simulink model "simulasi_dual-axis tracker"  (R2022b)
settings: Solver=VariableStepAuto  StartTime=0.0  StopTime=20  RelTol=1e-3
values from neighbouring files (symbols this model uses):
  a = Cx/Ap    (= 93255.7445539)    [parameter.m]
  b = 1/(W)^2    (= 0.000296140802632)    [parameter.m]
  c = 2*z/W    (= 0.057133023576)    [parameter.m]
  d = 1    [parameter.m]    (also in sun_calculation.m = datetime('now','TimeZone','UTC+7','Format','dd/MM/yyyy HH:mm)
  k = 150    [parameter.m]
  Kc = 1.3    [parameter.m]
  L = 0.98    [parameter.m]
  m = 0.01    [parameter.m]
  R = 230.77    [parameter.m]
libraries: fuzblock x16
settings Model: Creator=HP  LastModifiedBy=HP

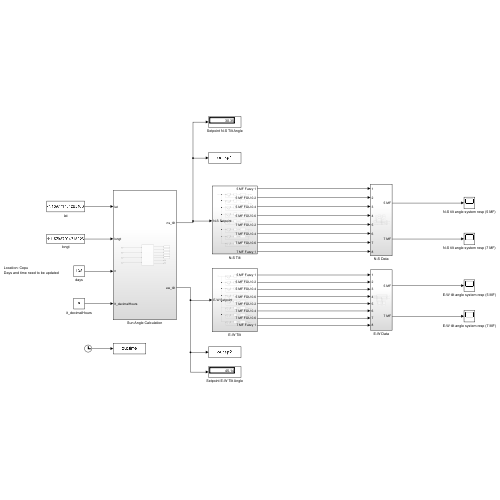
[thumbnail: Simulink's stored preview of the top-level diagram]
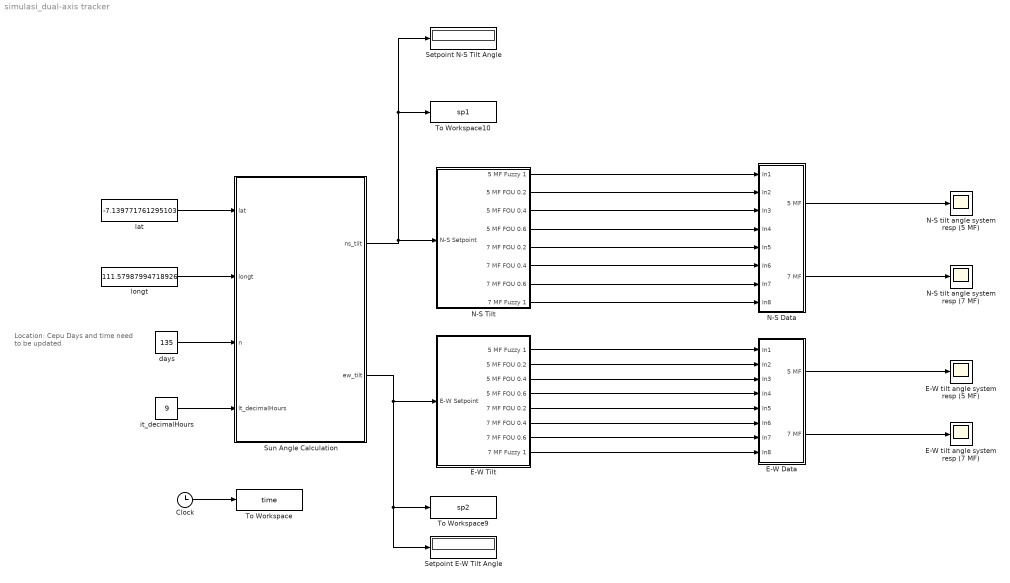
== system simulasi_dual-axis tracker ==
  note: Location: Cepu
      | Days and time need to be updated
  Clock : Clock
  E-W Data : Subsystem
  E-W Tilt : Subsystem
  E-W tilt angle system resp (5 MF) : Scope
  E-W tilt angle system resp (7 MF) : Scope
  N-S Data : Subsystem
  N-S Tilt : Subsystem
  N-S tilt angle system resp (5 MF) : Scope
  N-S tilt angle system resp (7 MF) : Scope
  Setpoint E-W Tilt Angle : Display
  Setpoint N-S Tilt Angle : Display
  Sun Angle Calculation : Subsystem
  To Workspace : ToWorkspace  VariableName=time  SampleTime=-1
  To Workspace10 : ToWorkspace  VariableName=sp1  SampleTime=-1
  To Workspace9 : ToWorkspace  VariableName=sp2  SampleTime=-1
  days : Constant  Value=135
  it_decimalHours : Constant  Value=9
  lat : Constant  Value=-7.139771761295103
  longt : Constant  Value=111.57987994718926
  wires:
  days/1 -> Sun Angle Calculation/3(n)
  longt/1 -> Sun Angle Calculation/2(longt)
  lat/1 -> Sun Angle Calculation/1(lat)
  it_decimalHours/1 -> Sun Angle Calculation/4(lt_decimalHours)
  Clock/1 -> To Workspace/1
  Sun Angle Calculation/1(ns_tilt) -> To Workspace10/1, Setpoint N-S Tilt Angle/1, N-S Tilt/1(N-S Setpoint)
  Sun Angle Calculation/2(ew_tilt) -> E-W Tilt/1(E-W Setpoint), Setpoint E-W Tilt Angle/1, To Workspace9/1
  E-W Tilt/1(5 MF Fuzzy 1) -> E-W Data/1(In1)
  E-W Tilt/2(5 MF FOU 0.2) -> E-W Data/2(In2)
  E-W Tilt/3(5 MF FOU 0.4) -> E-W Data/3(In3)
  E-W Tilt/4(5 MF FOU 0.6) -> E-W Data/4(In4)
  E-W Tilt/5(7 MF FOU 0.2) -> E-W Data/5(In5)
  E-W Tilt/6(7 MF FOU 0.4) -> E-W Data/6(In6)
  E-W Tilt/7(7 MF FOU 0.6) -> E-W Data/7(In7)
  E-W Tilt/8(7 MF Fuzzy 1) -> E-W Data/8(In8)
  E-W Data/1(5 MF) -> E-W tilt angle system resp (5 MF)/1
  E-W Data/2(7 MF) -> E-W tilt angle system resp (7 MF)/1
  N-S Tilt/1(5 MF Fuzzy 1) -> N-S Data/1(In1)
  N-S Tilt/2(5 MF FOU 0.2) -> N-S Data/2(In2)
  N-S Tilt/3(5 MF FOU 0.4) -> N-S Data/3(In3)
  N-S Tilt/4(5 MF FOU 0.6) -> N-S Data/4(In4)
  N-S Tilt/5(7 MF FOU 0.2) -> N-S Data/5(In5)
  N-S Tilt/6(7 MF FOU 0.4) -> N-S Data/6(In6)
  N-S Tilt/7(7 MF FOU 0.6) -> N-S Data/7(In7)
  N-S Tilt/8(7 MF Fuzzy 1) -> N-S Data/8(In8)
  N-S Data/1(5 MF) -> N-S tilt angle system resp (5 MF)/1
  N-S Data/2(7 MF) -> N-S tilt angle system resp (7 MF)/1

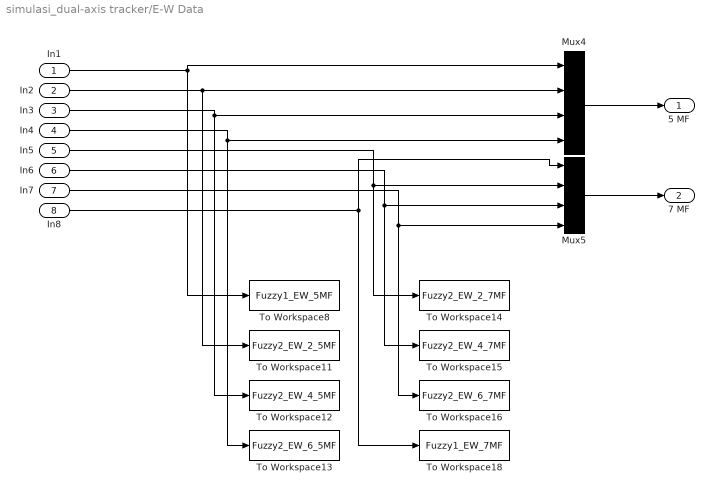
== system simulasi_dual-axis tracker/E-W Data ==
  In1 : Inport
  In2 : Inport  Port=2
  In3 : Inport  Port=3
  In4 : Inport  Port=4
  In5 : Inport  Port=5
  In6 : Inport  Port=6
  In7 : Inport  Port=7
  In8 : Inport  Port=8
  Mux4 : Mux
  Mux5 : Mux
  To Workspace11 : ToWorkspace  VariableName=Fuzzy2_EW_2_5MF  SampleTime=-1
  To Workspace12 : ToWorkspace  VariableName=Fuzzy2_EW_4_5MF  SampleTime=-1
  To Workspace13 : ToWorkspace  VariableName=Fuzzy2_EW_6_5MF  SampleTime=-1
  To Workspace14 : ToWorkspace  VariableName=Fuzzy2_EW_2_7MF  SampleTime=-1
  To Workspace15 : ToWorkspace  VariableName=Fuzzy2_EW_4_7MF  SampleTime=-1
  To Workspace16 : ToWorkspace  VariableName=Fuzzy2_EW_6_7MF  SampleTime=-1
  To Workspace18 : ToWorkspace  VariableName=Fuzzy1_EW_7MF  SampleTime=-1
  To Workspace8 : ToWorkspace  VariableName=Fuzzy1_EW_5MF  SampleTime=-1
  5 MF : Outport
  7 MF : Outport  Port=2
  wires:
  In7/1 -> To Workspace16/1, Mux5/4
  In4/1 -> To Workspace13/1, Mux4/4
  In6/1 -> To Workspace15/1, Mux5/3
  In1/1 -> Mux4/1, To Workspace8/1
  In8/1 -> Mux5/1, To Workspace18/1
  In2/1 -> To Workspace11/1, Mux4/2
  In5/1 -> To Workspace14/1, Mux5/2
  In3/1 -> To Workspace12/1, Mux4/3
  Mux4/1 -> 5 MF/1
  Mux5/1 -> 7 MF/1

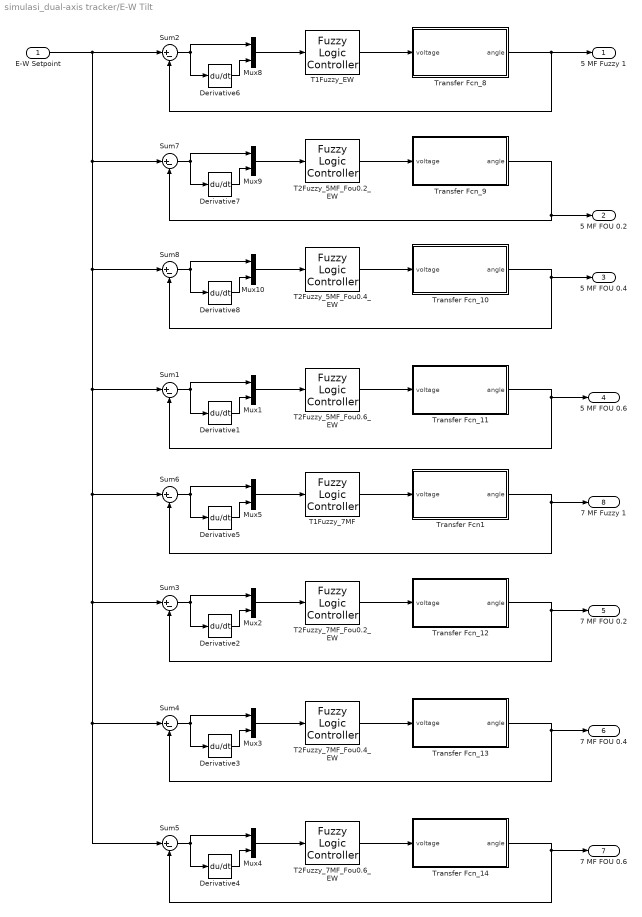
== system simulasi_dual-axis tracker/E-W Tilt ==
  E-W Setpoint : Inport
  Derivative{1..8} (8 alike) : Derivative
  Mux{1..5,8..10} (8 alike) : Mux  Inputs=2
  Sum{1..8} (8 alike) : Sum  Inputs=|+-
  T1Fuzzy_7MF : fuzblock/Fuzzy Logic  Controller  FIS='7mf_type1.fis'  OutputSampleNumber=101  DataType=double  FuzzifiedInputs=off  RuleFiringStrengths=off  RuleOutputs=off  AggregatedOutputs=off  SimulateUsing=Interpreted execution  OutOfRangeInputValueMessage=warning  NoRuleFiredMessage=warning  EmptyOutputFuzzySetMessage=warning
  T1Fuzzy_EW : fuzblock/Fuzzy Logic  Controller  FIS='5mf_type1.fis'  OutputSampleNumber=101  DataType=double  FuzzifiedInputs=off  RuleFiringStrengths=off  RuleOutputs=off  AggregatedOutputs=off  SimulateUsing=Interpreted execution  OutOfRangeInputValueMessage=warning  NoRuleFiredMessage=warning  EmptyOutputFuzzySetMessage=warning
  T2Fuzzy_5MF_Fou0.2_EW : fuzblock/Fuzzy Logic  Controller  FIS='5mf_type2_fou0.2.fis'  OutputSampleNumber=101  DataType=double  FuzzifiedInputs=off  RuleFiringStrengths=off  RuleOutputs=off  AggregatedOutputs=off  SimulateUsing=Interpreted execution  OutOfRangeInputValueMessage=warning  NoRuleFiredMessage=warning  EmptyOutputFuzzySetMessage=warning
  T2Fuzzy_5MF_Fou0.4_EW : fuzblock/Fuzzy Logic  Controller  FIS='5mf_type2_fou0.4.fis'  OutputSampleNumber=101  DataType=double  FuzzifiedInputs=off  RuleFiringStrengths=off  RuleOutputs=off  AggregatedOutputs=off  SimulateUsing=Interpreted execution  OutOfRangeInputValueMessage=warning  NoRuleFiredMessage=warning  EmptyOutputFuzzySetMessage=warning
  T2Fuzzy_5MF_Fou0.6_EW : fuzblock/Fuzzy Logic  Controller  FIS='5mf_type2_fou0.6.fis'  OutputSampleNumber=101  DataType=double  FuzzifiedInputs=off  RuleFiringStrengths=off  RuleOutputs=off  AggregatedOutputs=off  SimulateUsing=Interpreted execution  OutOfRangeInputValueMessage=warning  NoRuleFiredMessage=warning  EmptyOutputFuzzySetMessage=warning
  T2Fuzzy_7MF_Fou0.2_EW : fuzblock/Fuzzy Logic  Controller  FIS='7mf_type2_fou0.2.fis'  OutputSampleNumber=101  DataType=double  FuzzifiedInputs=off  RuleFiringStrengths=off  RuleOutputs=off  AggregatedOutputs=off  SimulateUsing=Interpreted execution  OutOfRangeInputValueMessage=warning  NoRuleFiredMessage=warning  EmptyOutputFuzzySetMessage=warning
  T2Fuzzy_7MF_Fou0.4_EW : fuzblock/Fuzzy Logic  Controller  FIS='7mf_type2_fou0.4.fis'  OutputSampleNumber=101  DataType=double  FuzzifiedInputs=off  RuleFiringStrengths=off  RuleOutputs=off  AggregatedOutputs=off  SimulateUsing=Interpreted execution  OutOfRangeInputValueMessage=warning  NoRuleFiredMessage=warning  EmptyOutputFuzzySetMessage=warning
  T2Fuzzy_7MF_Fou0.6_EW : fuzblock/Fuzzy Logic  Controller  FIS='7mf_type2_fou0.6.fis'  OutputSampleNumber=101  DataType=double  FuzzifiedInputs=off  RuleFiringStrengths=off  RuleOutputs=off  AggregatedOutputs=off  SimulateUsing=Interpreted execution  OutOfRangeInputValueMessage=warning  NoRuleFiredMessage=warning  EmptyOutputFuzzySetMessage=warning
  Transfer Fcn1 : Subsystem
  Transfer Fcn_10 : Subsystem
  Transfer Fcn_11 : Subsystem
  Transfer Fcn_12 : Subsystem
  Transfer Fcn_13 : Subsystem
  Transfer Fcn_14 : Subsystem
  Transfer Fcn_8 : Subsystem
  Transfer Fcn_9 : Subsystem
  5 MF Fuzzy 1 : Outport
  5 MF FOU 0.2 : Outport  Port=2
  5 MF FOU 0.4 : Outport  Port=3
  5 MF FOU 0.6 : Outport  Port=4
  7 MF FOU 0.2 : Outport  Port=5
  7 MF FOU 0.4 : Outport  Port=6
  7 MF FOU 0.6 : Outport  Port=7
  7 MF Fuzzy 1 : Outport  Port=8
  wires:
  Sum7/1 -> Derivative7/1, Mux9/1
  Transfer Fcn_9/1(angle) -> 5 MF FOU 0.2/1, Sum7/2
  T2Fuzzy_5MF_Fou0.4_EW/1 -> Transfer Fcn_10/1(voltage)
  Transfer Fcn_10/1(angle) -> 5 MF FOU 0.4/1, Sum8/2
  Derivative7/1 -> Mux9/2
  Mux9/1 -> T2Fuzzy_5MF_Fou0.2_EW/1
  Mux10/1 -> T2Fuzzy_5MF_Fou0.4_EW/1
  Derivative6/1 -> Mux8/2
  Mux8/1 -> T1Fuzzy_EW/1
  Sum2/1 -> Derivative6/1, Mux8/1
  Sum8/1 -> Derivative8/1, Mux10/1
  Derivative8/1 -> Mux10/2
  T1Fuzzy_EW/1 -> Transfer Fcn_8/1(voltage)
  Transfer Fcn_8/1(angle) -> 5 MF Fuzzy 1/1, Sum2/2
  T2Fuzzy_5MF_Fou0.2_EW/1 -> Transfer Fcn_9/1(voltage)
  Derivative1/1 -> Mux1/2
  Sum1/1 -> Derivative1/1, Mux1/1
  Mux1/1 -> T2Fuzzy_5MF_Fou0.6_EW/1
  Transfer Fcn_11/1(angle) -> 5 MF FOU 0.6/1, Sum1/2
  T2Fuzzy_5MF_Fou0.6_EW/1 -> Transfer Fcn_11/1(voltage)
  Sum3/1 -> Derivative2/1, Mux2/1
  Mux2/1 -> T2Fuzzy_7MF_Fou0.2_EW/1
  Derivative2/1 -> Mux2/2
  T2Fuzzy_7MF_Fou0.2_EW/1 -> Transfer Fcn_12/1(voltage)
  Transfer Fcn_12/1(angle) -> 7 MF FOU 0.2/1, Sum3/2
  Mux3/1 -> T2Fuzzy_7MF_Fou0.4_EW/1
  Sum4/1 -> Derivative3/1, Mux3/1
  Transfer Fcn_13/1(angle) -> 7 MF FOU 0.4/1, Sum4/2
  Derivative3/1 -> Mux3/2
  T2Fuzzy_7MF_Fou0.4_EW/1 -> Transfer Fcn_13/1(voltage)
  T2Fuzzy_7MF_Fou0.6_EW/1 -> Transfer Fcn_14/1(voltage)
  Derivative4/1 -> Mux4/2
  Sum5/1 -> Derivative4/1, Mux4/1
  Transfer Fcn_14/1(angle) -> 7 MF FOU 0.6/1, Sum5/2
  Mux4/1 -> T2Fuzzy_7MF_Fou0.6_EW/1
  Transfer Fcn1/1(angle) -> 7 MF Fuzzy 1/1, Sum6/2
  E-W Setpoint/1 -> Sum6/1, Sum5/1, Sum4/1, Sum3/1, Sum1/1, Sum8/1, Sum7/1, Sum2/1
  Derivative5/1 -> Mux5/2
  Mux5/1 -> T1Fuzzy_7MF/1
  Sum6/1 -> Derivative5/1, Mux5/1
  T1Fuzzy_7MF/1 -> Transfer Fcn1/1(voltage)

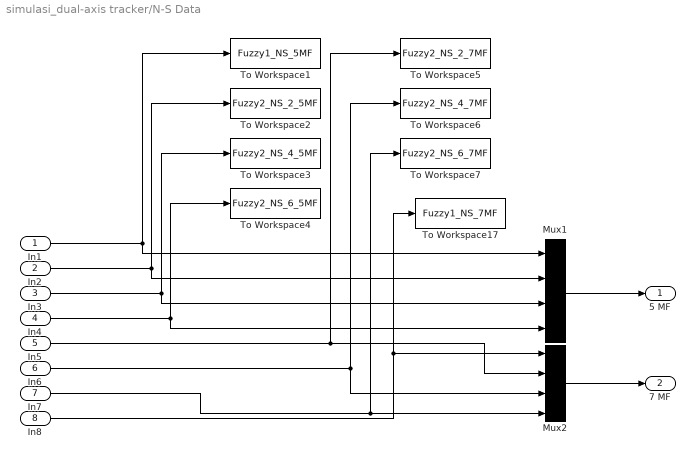
== system simulasi_dual-axis tracker/N-S Data ==
  In1 : Inport
  In2 : Inport  Port=2
  In3 : Inport  Port=3
  In4 : Inport  Port=4
  In5 : Inport  Port=5
  In6 : Inport  Port=6
  In7 : Inport  Port=7
  In8 : Inport  Port=8
  Mux1 : Mux
  Mux2 : Mux
  To Workspace1 : ToWorkspace  VariableName=Fuzzy1_NS_5MF  SampleTime=-1
  To Workspace17 : ToWorkspace  VariableName=Fuzzy1_NS_7MF  SampleTime=-1
  To Workspace2 : ToWorkspace  VariableName=Fuzzy2_NS_2_5MF  SampleTime=-1
  To Workspace3 : ToWorkspace  VariableName=Fuzzy2_NS_4_5MF  SampleTime=-1
  To Workspace4 : ToWorkspace  VariableName=Fuzzy2_NS_6_5MF  SampleTime=-1
  To Workspace5 : ToWorkspace  VariableName=Fuzzy2_NS_2_7MF  SampleTime=-1
  To Workspace6 : ToWorkspace  VariableName=Fuzzy2_NS_4_7MF  SampleTime=-1
  To Workspace7 : ToWorkspace  VariableName=Fuzzy2_NS_6_7MF  SampleTime=-1
  5 MF : Outport
  7 MF : Outport  Port=2
  wires:
  In8/1 -> To Workspace17/1, Mux2/1
  In2/1 -> Mux1/2, To Workspace2/1
  In5/1 -> Mux2/2, To Workspace5/1
  In6/1 -> Mux2/3, To Workspace6/1
  In3/1 -> Mux1/3, To Workspace3/1
  In4/1 -> Mux1/4, To Workspace4/1
  In7/1 -> To Workspace7/1, Mux2/4
  In1/1 -> Mux1/1, To Workspace1/1
  Mux1/1 -> 5 MF/1
  Mux2/1 -> 7 MF/1

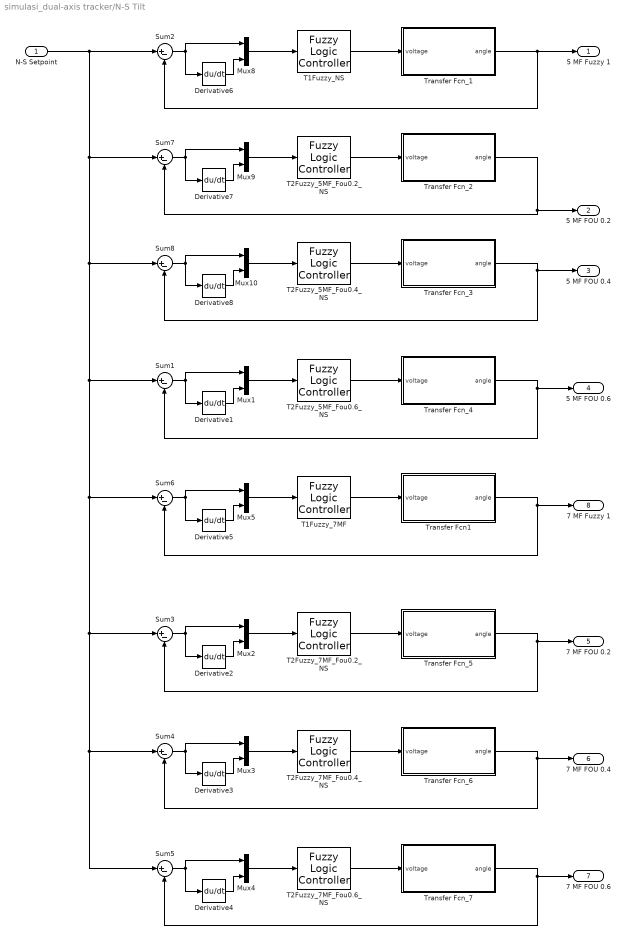
== system simulasi_dual-axis tracker/N-S Tilt ==
  N-S Setpoint : Inport
  Derivative{1..8} (8 alike) : Derivative
  Mux{1..5,8..10} (8 alike) : Mux  Inputs=2
  Sum{1..8} (8 alike) : Sum  Inputs=|+-
  T1Fuzzy_7MF : fuzblock/Fuzzy Logic  Controller  FIS='7mf_type1.fis'  OutputSampleNumber=101  DataType=double  FuzzifiedInputs=off  RuleFiringStrengths=off  RuleOutputs=off  AggregatedOutputs=off  SimulateUsing=Interpreted execution  OutOfRangeInputValueMessage=warning  NoRuleFiredMessage=warning  EmptyOutputFuzzySetMessage=warning
  T1Fuzzy_NS : fuzblock/Fuzzy Logic  Controller  FIS='5mf_type1.fis'  OutputSampleNumber=101  DataType=double  FuzzifiedInputs=off  RuleFiringStrengths=off  RuleOutputs=off  AggregatedOutputs=off  SimulateUsing=Interpreted execution  OutOfRangeInputValueMessage=warning  NoRuleFiredMessage=warning  EmptyOutputFuzzySetMessage=warning
  T2Fuzzy_5MF_Fou0.2_NS : fuzblock/Fuzzy Logic  Controller  FIS='5mf_type2_fou0.2.fis'  OutputSampleNumber=101  DataType=double  FuzzifiedInputs=off  RuleFiringStrengths=off  RuleOutputs=off  AggregatedOutputs=off  SimulateUsing=Interpreted execution  OutOfRangeInputValueMessage=warning  NoRuleFiredMessage=warning  EmptyOutputFuzzySetMessage=warning
  T2Fuzzy_5MF_Fou0.4_NS : fuzblock/Fuzzy Logic  Controller  FIS='5mf_type2_fou0.4.fis'  OutputSampleNumber=101  DataType=double  FuzzifiedInputs=off  RuleFiringStrengths=off  RuleOutputs=off  AggregatedOutputs=off  SimulateUsing=Interpreted execution  OutOfRangeInputValueMessage=warning  NoRuleFiredMessage=warning  EmptyOutputFuzzySetMessage=warning
  T2Fuzzy_5MF_Fou0.6_NS : fuzblock/Fuzzy Logic  Controller  FIS='5mf_type2_fou0.6.fis'  OutputSampleNumber=101  DataType=double  FuzzifiedInputs=off  RuleFiringStrengths=off  RuleOutputs=off  AggregatedOutputs=off  SimulateUsing=Interpreted execution  OutOfRangeInputValueMessage=warning  NoRuleFiredMessage=warning  EmptyOutputFuzzySetMessage=warning
  T2Fuzzy_7MF_Fou0.2_NS : fuzblock/Fuzzy Logic  Controller  FIS='7mf_type2_fou0.2.fis'  OutputSampleNumber=101  DataType=double  FuzzifiedInputs=off  RuleFiringStrengths=off  RuleOutputs=off  AggregatedOutputs=off  SimulateUsing=Interpreted execution  OutOfRangeInputValueMessage=warning  NoRuleFiredMessage=warning  EmptyOutputFuzzySetMessage=warning
  T2Fuzzy_7MF_Fou0.4_NS : fuzblock/Fuzzy Logic  Controller  FIS='7mf_type2_fou0.4.fis'  OutputSampleNumber=101  DataType=double  FuzzifiedInputs=off  RuleFiringStrengths=off  RuleOutputs=off  AggregatedOutputs=off  SimulateUsing=Interpreted execution  OutOfRangeInputValueMessage=warning  NoRuleFiredMessage=warning  EmptyOutputFuzzySetMessage=warning
  T2Fuzzy_7MF_Fou0.6_NS : fuzblock/Fuzzy Logic  Controller  FIS='7mf_type2_fou0.6.fis'  OutputSampleNumber=101  DataType=double  FuzzifiedInputs=off  RuleFiringStrengths=off  RuleOutputs=off  AggregatedOutputs=off  SimulateUsing=Interpreted execution  OutOfRangeInputValueMessage=warning  NoRuleFiredMessage=warning  EmptyOutputFuzzySetMessage=warning
  Transfer Fcn1 : Subsystem
  Transfer Fcn_1 : Subsystem
  Transfer Fcn_2 : Subsystem
  Transfer Fcn_3 : Subsystem
  Transfer Fcn_4 : Subsystem
  Transfer Fcn_5 : Subsystem
  Transfer Fcn_6 : Subsystem
  Transfer Fcn_7 : Subsystem
  5 MF Fuzzy 1 : Outport
  5 MF FOU 0.2 : Outport  Port=2
  5 MF FOU 0.4 : Outport  Port=3
  5 MF FOU 0.6 : Outport  Port=4
  7 MF FOU 0.2 : Outport  Port=5
  7 MF FOU 0.4 : Outport  Port=6
  7 MF FOU 0.6 : Outport  Port=7
  7 MF Fuzzy 1 : Outport  Port=8
  wires:
  Derivative3/1 -> Mux3/2
  Transfer Fcn_4/1(angle) -> 5 MF FOU 0.6/1, Sum1/2
  Transfer Fcn_7/1(angle) -> 7 MF FOU 0.6/1, Sum5/2
  T2Fuzzy_7MF_Fou0.6_NS/1 -> Transfer Fcn_7/1(voltage)
  Mux4/1 -> T2Fuzzy_7MF_Fou0.6_NS/1
  Derivative8/1 -> Mux10/2
  Transfer Fcn_3/1(angle) -> 5 MF FOU 0.4/1, Sum8/2
  Derivative2/1 -> Mux2/2
  Sum7/1 -> Derivative7/1, Mux9/1
  Sum3/1 -> Derivative2/1, Mux2/1
  Transfer Fcn_1/1(angle) -> 5 MF Fuzzy 1/1, Sum2/2
  Mux9/1 -> T2Fuzzy_5MF_Fou0.2_NS/1
  Mux2/1 -> T2Fuzzy_7MF_Fou0.2_NS/1
  Sum5/1 -> Derivative4/1, Mux4/1
  T2Fuzzy_5MF_Fou0.6_NS/1 -> Transfer Fcn_4/1(voltage)
  Derivative6/1 -> Mux8/2
  Sum2/1 -> Derivative6/1, Mux8/1
  Sum8/1 -> Derivative8/1, Mux10/1
  T2Fuzzy_5MF_Fou0.2_NS/1 -> Transfer Fcn_2/1(voltage)
  Transfer Fcn_5/1(angle) -> 7 MF FOU 0.2/1, Sum3/2
  Sum1/1 -> Derivative1/1, Mux1/1
  Mux3/1 -> T2Fuzzy_7MF_Fou0.4_NS/1
  Mux8/1 -> T1Fuzzy_NS/1
  Mux1/1 -> T2Fuzzy_5MF_Fou0.6_NS/1
  Derivative1/1 -> Mux1/2
  Derivative4/1 -> Mux4/2
  Transfer Fcn_2/1(angle) -> 5 MF FOU 0.2/1, Sum7/2
  Derivative7/1 -> Mux9/2
  Mux10/1 -> T2Fuzzy_5MF_Fou0.4_NS/1
  T1Fuzzy_NS/1 -> Transfer Fcn_1/1(voltage)
  T2Fuzzy_7MF_Fou0.2_NS/1 -> Transfer Fcn_5/1(voltage)
  T2Fuzzy_5MF_Fou0.4_NS/1 -> Transfer Fcn_3/1(voltage)
  Transfer Fcn_6/1(angle) -> 7 MF FOU 0.4/1, Sum4/2
  Sum4/1 -> Derivative3/1, Mux3/1
  T2Fuzzy_7MF_Fou0.4_NS/1 -> Transfer Fcn_6/1(voltage)
  N-S Setpoint/1 -> Sum6/1, Sum5/1, Sum4/1, Sum3/1, Sum1/1, Sum8/1, Sum7/1, Sum2/1
  Mux5/1 -> T1Fuzzy_7MF/1
  Transfer Fcn1/1(angle) -> 7 MF Fuzzy 1/1, Sum6/2
  Sum6/1 -> Derivative5/1, Mux5/1
  Derivative5/1 -> Mux5/2
  T1Fuzzy_7MF/1 -> Transfer Fcn1/1(voltage)

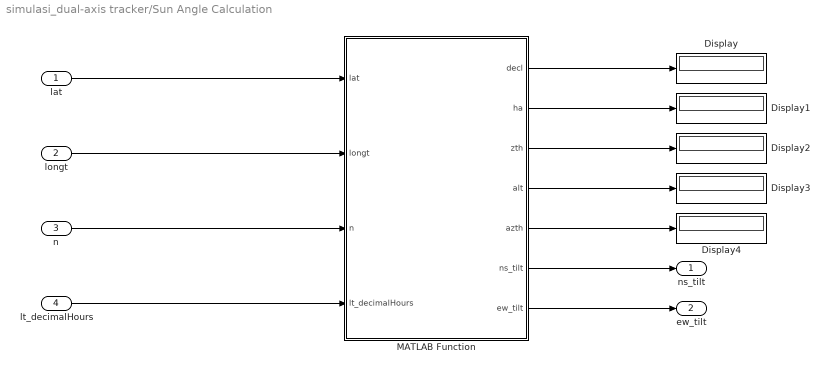
== system simulasi_dual-axis tracker/Sun Angle Calculation ==
  lat : Inport
  longt : Inport  Port=2
  n : Inport  Port=3
  lt_decimalHours : Inport  Port=4
  Display{,1..4} (5 alike) : Display
  MATLAB Function : MATLAB Function  TreatAsAtomicUnit=on
  ns_tilt : Outport
  ew_tilt : Outport  Port=2
  wires:
  MATLAB Function/4(alt) -> Display3/1
  MATLAB Function/2(ha) -> Display1/1
  n/1 -> MATLAB Function/3(n)
  MATLAB Function/3(zth) -> Display2/1
  MATLAB Function/5(azth) -> Display4/1
  MATLAB Function/6(ns_tilt) -> ns_tilt/1
  lt_decimalHours/1 -> MATLAB Function/4(lt_decimalHours)
  MATLAB Function/1(decl) -> Display/1
  longt/1 -> MATLAB Function/2(longt)
  lat/1 -> MATLAB Function/1(lat)
  MATLAB Function/7(ew_tilt) -> ew_tilt/1

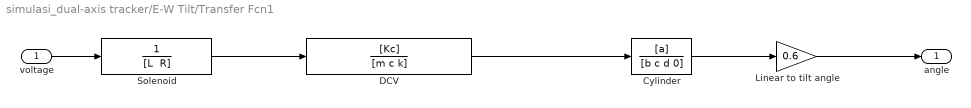
== system simulasi_dual-axis tracker/E-W Tilt/Transfer Fcn1 ==
  voltage : Inport
  Cylinder : TransferFcn  Numerator=[a]  Denominator=[b c d 0]
  DCV : TransferFcn  Numerator=[Kc]  Denominator=[m c k]
  Linear to tilt angle : Gain  Gain=0.6
  Solenoid : TransferFcn  Denominator="[L  R]"
  angle : Outport
  wires:
  Solenoid/1 -> DCV/1
  voltage/1 -> Solenoid/1
  DCV/1 -> Cylinder/1
  Cylinder/1 -> Linear to tilt angle/1
  Linear to tilt angle/1 -> angle/1

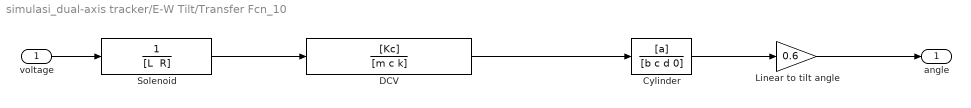
== system simulasi_dual-axis tracker/E-W Tilt/Transfer Fcn_10 ==
  voltage : Inport
  Cylinder : TransferFcn  Numerator=[a]  Denominator=[b c d 0]
  DCV : TransferFcn  Numerator=[Kc]  Denominator=[m c k]
  Linear to tilt angle : Gain  Gain=0.6
  Solenoid : TransferFcn  Denominator="[L  R]"
  angle : Outport
  wires:
  Solenoid/1 -> DCV/1
  voltage/1 -> Solenoid/1
  DCV/1 -> Cylinder/1
  Cylinder/1 -> Linear to tilt angle/1
  Linear to tilt angle/1 -> angle/1

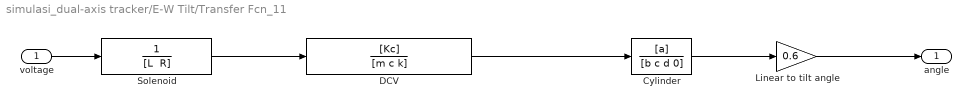
== system simulasi_dual-axis tracker/E-W Tilt/Transfer Fcn_11 ==
  voltage : Inport
  Cylinder : TransferFcn  Numerator=[a]  Denominator=[b c d 0]
  DCV : TransferFcn  Numerator=[Kc]  Denominator=[m c k]
  Linear to tilt angle : Gain  Gain=0.6
  Solenoid : TransferFcn  Denominator="[L  R]"
  angle : Outport
  wires:
  Solenoid/1 -> DCV/1
  voltage/1 -> Solenoid/1
  DCV/1 -> Cylinder/1
  Cylinder/1 -> Linear to tilt angle/1
  Linear to tilt angle/1 -> angle/1

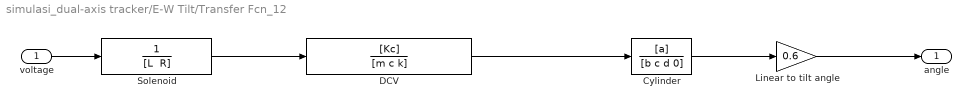
== system simulasi_dual-axis tracker/E-W Tilt/Transfer Fcn_12 ==
  voltage : Inport
  Cylinder : TransferFcn  Numerator=[a]  Denominator=[b c d 0]
  DCV : TransferFcn  Numerator=[Kc]  Denominator=[m c k]
  Linear to tilt angle : Gain  Gain=0.6
  Solenoid : TransferFcn  Denominator="[L  R]"
  angle : Outport
  wires:
  Solenoid/1 -> DCV/1
  voltage/1 -> Solenoid/1
  DCV/1 -> Cylinder/1
  Cylinder/1 -> Linear to tilt angle/1
  Linear to tilt angle/1 -> angle/1

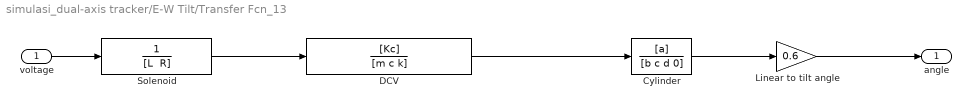
== system simulasi_dual-axis tracker/E-W Tilt/Transfer Fcn_13 ==
  voltage : Inport
  Cylinder : TransferFcn  Numerator=[a]  Denominator=[b c d 0]
  DCV : TransferFcn  Numerator=[Kc]  Denominator=[m c k]
  Linear to tilt angle : Gain  Gain=0.6
  Solenoid : TransferFcn  Denominator="[L  R]"
  angle : Outport
  wires:
  Solenoid/1 -> DCV/1
  voltage/1 -> Solenoid/1
  DCV/1 -> Cylinder/1
  Cylinder/1 -> Linear to tilt angle/1
  Linear to tilt angle/1 -> angle/1

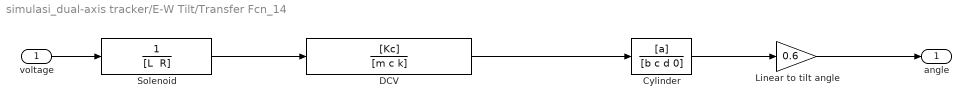
== system simulasi_dual-axis tracker/E-W Tilt/Transfer Fcn_14 ==
  voltage : Inport
  Cylinder : TransferFcn  Numerator=[a]  Denominator=[b c d 0]
  DCV : TransferFcn  Numerator=[Kc]  Denominator=[m c k]
  Linear to tilt angle : Gain  Gain=0.6
  Solenoid : TransferFcn  Denominator="[L  R]"
  angle : Outport
  wires:
  Solenoid/1 -> DCV/1
  voltage/1 -> Solenoid/1
  DCV/1 -> Cylinder/1
  Cylinder/1 -> Linear to tilt angle/1
  Linear to tilt angle/1 -> angle/1

== system simulasi_dual-axis tracker/E-W Tilt/Transfer Fcn_8 ==
  voltage : Inport
  Cylinder : TransferFcn  Numerator=[a]  Denominator=[b c d 0]
  DCV : TransferFcn  Numerator=[Kc]  Denominator=[m c k]
  Linear to tilt angle : Gain  Gain=0.6
  Solenoid : TransferFcn  Denominator="[L  R]"
  angle : Outport
  wires:
  Solenoid/1 -> DCV/1
  voltage/1 -> Solenoid/1
  DCV/1 -> Cylinder/1
  Cylinder/1 -> Linear to tilt angle/1
  Linear to tilt angle/1 -> angle/1

== system simulasi_dual-axis tracker/E-W Tilt/Transfer Fcn_9 ==
  voltage : Inport
  Cylinder : TransferFcn  Numerator=[a]  Denominator=[b c d 0]
  DCV : TransferFcn  Numerator=[Kc]  Denominator=[m c k]
  Linear to tilt angle : Gain  Gain=0.6
  Solenoid : TransferFcn  Denominator="[L  R]"
  angle : Outport
  wires:
  Solenoid/1 -> DCV/1
  voltage/1 -> Solenoid/1
  DCV/1 -> Cylinder/1
  Cylinder/1 -> Linear to tilt angle/1
  Linear to tilt angle/1 -> angle/1

== system simulasi_dual-axis tracker/N-S Tilt/Transfer Fcn1 ==
  voltage : Inport
  Cylinder : TransferFcn  Numerator=[a]  Denominator=[b c d 0]
  DCV : TransferFcn  Numerator=[Kc]  Denominator=[m c k]
  Linear to tilt angle : Gain  Gain=0.6
  Solenoid : TransferFcn  Denominator="[L  R]"
  angle : Outport
  wires:
  Solenoid/1 -> DCV/1
  voltage/1 -> Solenoid/1
  DCV/1 -> Cylinder/1
  Cylinder/1 -> Linear to tilt angle/1
  Linear to tilt angle/1 -> angle/1

== system simulasi_dual-axis tracker/N-S Tilt/Transfer Fcn_1 ==
  voltage : Inport
  Cylinder : TransferFcn  Numerator=[a]  Denominator=[b c d 0]
  DCV : TransferFcn  Numerator=[Kc]  Denominator=[m c k]
  Linear to tilt angle : Gain  Gain=0.6
  Solenoid : TransferFcn  Denominator="[L  R]"
  angle : Outport
  wires:
  Solenoid/1 -> DCV/1
  voltage/1 -> Solenoid/1
  DCV/1 -> Cylinder/1
  Cylinder/1 -> Linear to tilt angle/1
  Linear to tilt angle/1 -> angle/1

== system simulasi_dual-axis tracker/N-S Tilt/Transfer Fcn_2 ==
  voltage : Inport
  Cylinder : TransferFcn  Numerator=[a]  Denominator=[b c d 0]
  DCV : TransferFcn  Numerator=[Kc]  Denominator=[m c k]
  Linear to tilt angle : Gain  Gain=0.6
  Solenoid : TransferFcn  Denominator="[L  R]"
  angle : Outport
  wires:
  Solenoid/1 -> DCV/1
  voltage/1 -> Solenoid/1
  DCV/1 -> Cylinder/1
  Cylinder/1 -> Linear to tilt angle/1
  Linear to tilt angle/1 -> angle/1

== system simulasi_dual-axis tracker/N-S Tilt/Transfer Fcn_3 ==
  voltage : Inport
  Cylinder : TransferFcn  Numerator=[a]  Denominator=[b c d 0]
  DCV : TransferFcn  Numerator=[Kc]  Denominator=[m c k]
  Linear to tilt angle : Gain  Gain=0.6
  Solenoid : TransferFcn  Denominator="[L  R]"
  angle : Outport
  wires:
  Solenoid/1 -> DCV/1
  voltage/1 -> Solenoid/1
  DCV/1 -> Cylinder/1
  Cylinder/1 -> Linear to tilt angle/1
  Linear to tilt angle/1 -> angle/1

== system simulasi_dual-axis tracker/N-S Tilt/Transfer Fcn_4 ==
  voltage : Inport
  Cylinder : TransferFcn  Numerator=[a]  Denominator=[b c d 0]
  DCV : TransferFcn  Numerator=[Kc]  Denominator=[m c k]
  Linear to tilt angle : Gain  Gain=0.6
  Solenoid : TransferFcn  Denominator="[L  R]"
  angle : Outport
  wires:
  Solenoid/1 -> DCV/1
  voltage/1 -> Solenoid/1
  DCV/1 -> Cylinder/1
  Cylinder/1 -> Linear to tilt angle/1
  Linear to tilt angle/1 -> angle/1

== system simulasi_dual-axis tracker/N-S Tilt/Transfer Fcn_5 ==
  voltage : Inport
  Cylinder : TransferFcn  Numerator=[a]  Denominator=[b c d 0]
  DCV : TransferFcn  Numerator=[Kc]  Denominator=[m c k]
  Linear to tilt angle : Gain  Gain=0.6
  Solenoid : TransferFcn  Denominator="[L  R]"
  angle : Outport
  wires:
  Solenoid/1 -> DCV/1
  voltage/1 -> Solenoid/1
  DCV/1 -> Cylinder/1
  Cylinder/1 -> Linear to tilt angle/1
  Linear to tilt angle/1 -> angle/1

== system simulasi_dual-axis tracker/N-S Tilt/Transfer Fcn_6 ==
  voltage : Inport
  Cylinder : TransferFcn  Numerator=[a]  Denominator=[b c d 0]
  DCV : TransferFcn  Numerator=[Kc]  Denominator=[m c k]
  Linear to tilt angle : Gain  Gain=0.6
  Solenoid : TransferFcn  Denominator="[L  R]"
  angle : Outport
  wires:
  Solenoid/1 -> DCV/1
  voltage/1 -> Solenoid/1
  DCV/1 -> Cylinder/1
  Cylinder/1 -> Linear to tilt angle/1
  Linear to tilt angle/1 -> angle/1

== system simulasi_dual-axis tracker/N-S Tilt/Transfer Fcn_7 ==
  voltage : Inport
  Cylinder : TransferFcn  Numerator=[a]  Denominator=[b c d 0]
  DCV : TransferFcn  Numerator=[Kc]  Denominator=[m c k]
  Linear to tilt angle : Gain  Gain=0.6
  Solenoid : TransferFcn  Denominator="[L  R]"
  angle : Outport
  wires:
  Solenoid/1 -> DCV/1
  voltage/1 -> Solenoid/1
  DCV/1 -> Cylinder/1
  Cylinder/1 -> Linear to tilt angle/1
  Linear to tilt angle/1 -> angle/1

== matlab function simulasi_dual-axis tracker/Sun Angle Calculation/MATLAB Function ==
  data: lat input; decl output; longt input; n input; lt_decimalHours input; ha output; zth output; alt output; azth output; ns_tilt output; ew_tilt output
function [decl, ha, zth, alt, azth, ns_tilt, ew_tilt] = calculate_sun_angles(lat, longt, n, lt_decimalHours)

% Perhitungan Sudut Penjejak Matahari
% References: Karafil, et. al (2015)

% Declination Angle
decl = 23.45*sind((360*(284+n))/365);

% Hour Angle Calculation
T_utc = 7; % UTC zone for West Indonesia (Java, Sumatra, West Kalimantan)
LSTM = T_utc * 15; % local standard meridian time
B = 360/365 * (n-81); % calculate B parameter
eot = 9.87 * sind(2*B) - 7.53 * cosd(B) - 1.5 * sind(B); % equation of time
TC = 4 * (longt - LSTM) + eot; % time correction factor
lst = lt_decimalHours + TC/60; % calculate local solar time
ha = 15 * (lst - 12); % calculate hour angle

% Azimuth, Altitude, Zenith Angle
zth = acosd((sind(decl)*sind(lat))+(cosd(ha)*cosd(decl)*cosd(lat))); % zenith
alt = 90 - zth; % altitude/elevation    
if ha < 0 % azimuth if hour angle < 0
    azth = acosd((sind(decl)*cosd(lat)-cosd(decl)*sind(lat)*cosd(ha))/cosd(alt));
else % azimuth if hour angle > 0
    azth = 360 - acosd((sind(decl)*cosd(lat)-cosd(decl)*sind(lat)*cosd(ha))/cosd(alt));
end

% PV tilt angle
surf_azth = 0; % PV is headed north/due north
ns_tilt = atand(tand(zth)*abs(cosd(azth-surf_azth)));
ew_tilt = atand(tand(zth)*abs(cosd(surf_azth)));
